simulink model "Speed_Control_Of_Induction_Motor_SVPWM"  (R2023b)
settings: Solver=ode3  StartTime=0.0  StopTime=100  FixedStep=1e-5  RelTol=1e-3
undefined symbols (not defined in the file): DiscIntNeverNeededParam
libraries: spsIGBTDiodeLib x6, spsCurrentMeasurementLib x3, spsAsynchronousMachineSIUnitsLib x1, slpidlib x1, simulink x1, spsDCVoltageSourceLib x1, sps_lib x1
settings Model: Creator=mailb  LastModifiedBy=mailb

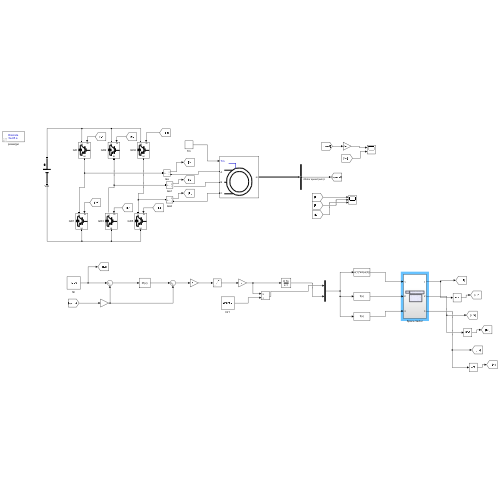
[thumbnail: Simulink's stored preview of the top-level diagram]
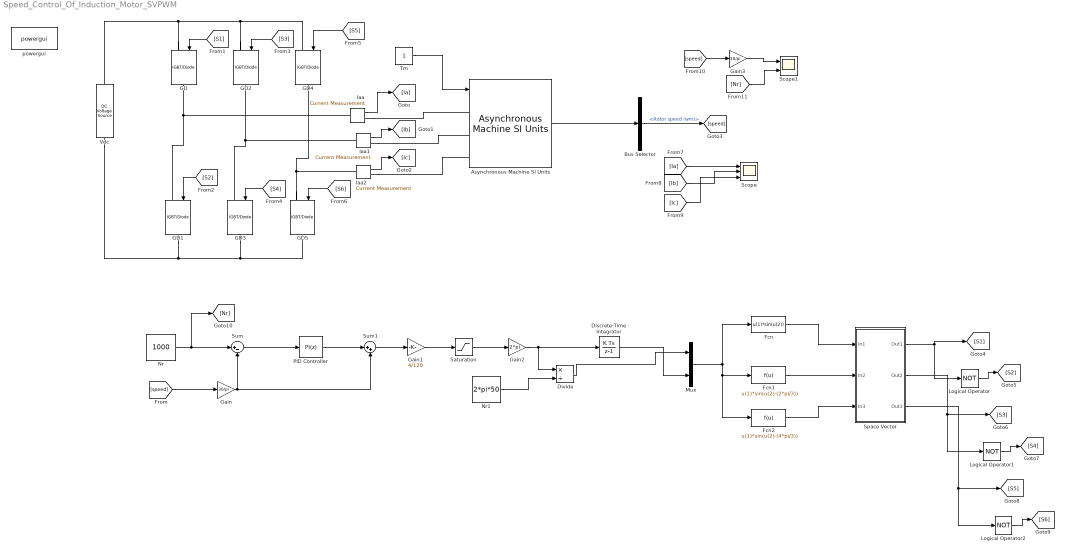
== system Speed_Control_Of_Induction_Motor_SVPWM ==
  Asynchronous Machine SI Units : spsAsynchronousMachineSIUnitsLib/Asynchronous Machine SI Units  RotorType=Squirrel-cage  PresetModel=No  MechanicalLoad=Torque Tm  ShowDetailedParameters=on  ReferenceFrame=Rotor  Units=SI  MeasurementBus=off  NominalParameters=[1.845e+04 400 50]  VoltageRatio=1  Stator=[0.5968 0.0003495]  Rotor=[0.6258 0.005473]  Cage1=[0.4155 0.002066]  Cage2=[0.4168 0.0003495]  Lm=0.0354  Mechanical=[0.05 0.005879 2]  PolePairs=2  InitialConditions=[0 0 0 0 0 0 0 0]  SimulateSaturation=off  Saturation=[14.03593122, 27.81365428, 53.79336849, 72.68890987, 97.98006896, 148.6815601, 215.7428561, 302.9841135, 428.7778367 ; 230, 322, 414, 460, 506, 552, 598, 644, 690]  LoadFlowParameters=1492000  TsPowergui=0  TsBlock=-1  IterativeModel=Trapezoidal non iterative  IterativeDiscreteModel=Trapezoidal non iterative  Pmec=1.492e+006
  Bus Selector : BusSelector  OutputSignals=Mechanical.Rotor speed (wm)
  Discrete-Time Integrator : DiscreteIntegrator  SampleTime=-1  ICPrevOutput=DiscIntNeverNeededParam  ICPrevScaledInput=DiscIntNeverNeededParam
  Divide : Product  Inputs=*/
  Fcn : Fcn  Expr=u(1)*sin(u(2))
  Fcn1 : Fcn  Expr=u(1)*sin(u(2)-(2*pi/3))
  Fcn2 : Fcn  Expr=u(1)*sin(u(2)-(4*pi/3))
  GD{,1..5} (6 alike) : spsIGBTDiodeLib/IGBT//Diode  Ron=1e-3  Rs=1e5  Cs=inf  Measurements=off
  Gain : Gain  Gain=30/pi
  Gain1 : Gain  Gain=4/120
  Gain2 : Gain  Gain=2*pi
  Gain3 : Gain  Gain=30/pi
  Iaa : spsCurrentMeasurementLib/Current Measurement  PhasorSimulation=off  OutputType=Complex  PSBequivalent=0
  Iaa1 : spsCurrentMeasurementLib/Current Measurement  PhasorSimulation=off  OutputType=Complex  PSBequivalent=0
  Iaa2 : spsCurrentMeasurementLib/Current Measurement  PhasorSimulation=off  OutputType=Complex  PSBequivalent=0
  Logical Operator : Logic  Operator=NOT  AllPortsSameDT=off  OutDataTypeStr=boolean
  Logical Operator1 : Logic  Operator=NOT  AllPortsSameDT=off  OutDataTypeStr=boolean
  Logical Operator2 : Logic  Operator=NOT  AllPortsSameDT=off  OutDataTypeStr=boolean
  Mux : Mux  Inputs=2
  Nr : Constant  Value=1000
  Nr1 : Constant  Value=2*pi*50
  PID Controller : slpidlib/PID Controller  Controller=PI  Form=Parallel  TimeDomain=Discrete-time  UseExternalTs=off  SampleTime=-1  IntegratorMethod=Forward Euler  FilterMethod=Forward Euler  ControllerParametersSource=internal  P=1  I=10  UseKiTs=off  D=0  N=100  UseFilter=on  TunerSelectOption=Transfer Function Based (PID Tuner App)  InitialConditionSource=internal  InitialConditionForIntegrator=0  InitialConditionForFilter=0  DifferentiatorICPrevScaledInput=0  ExternalReset=none  TrackingMode=off  Kt=1  LimitOutput=off  SatLimitsSource=internal  UpperSaturationLimit=inf  LowerSaturationLimit=-inf  LinearizeAsGain=on  AntiWindupMode=none  Kb=1  LimitIntegrator=off  UpperIntegratorSaturationLimit=inf  LowerIntegratorSaturationLimit=-inf  POutMin=[]  POutMax=[]  IOutMin=[]  IOutMax=[]  DOutMin=[]  DOutMax=[]  NOutMin=[]  NOutMax=[]  SumOutMin=[]  SumOutMax=[]  SaturationOutMin=[]  SaturationOutMax=[]  PParamMin=[]  PParamMax=[]  IParamMin=[]  IParamMax=[]  DParamMin=[]  DParamMax=[]  NParamMin=[]  NParamMax=[]  KbParamMin=[]  KbParamMax=[]  KtParamMin=[]  KtParamMax=[]  KbOutMin=[]  KbOutMax=[]  KtOutMin=[]  KtOutMax=[]  IntegratorOutMin=[]  IntegratorOutMax=[]  FilterOutMin=[]  FilterOutMax=[]  SumI1OutMin=[]  SumI1OutMax=[]  SumI2OutMin=[]  SumI2OutMax=[]  SumI3OutMin=[]  SumI3OutMax=[]  SumI4OutMin=[]  SumI4OutMax=[]  SumDOutMin=[]  SumDOutMax=[]  DifferentiatorOutMin=[]  DifferentiatorOutMax=[]  FilterDiffOutCoefMin=[]  FilterDiffOutCoefMax=[]  ReciprocalOutMin=[]  ReciprocalOutMax=[]  SumDenOutMin=[]  SumDenOutMax=[]  SumNumOutMin=[]  SumNumOutMax=[]  DivideOutMin=[]  DivideOutMax=[]  UdiffTsProdOutMin=[]  UdiffTsProdOutMax=[]  NTsProdOutMin=[]  NTsProdOutMax=[]  UintegralTsProdOutMin=[]  UintegralTsProdOutMax=[]  UngainTsProdOutMin=[]  UngainTsProdOutMax=[]  ClampingZeroOutDataTypeStr=Inherit: Inherit via back propagation  ClampingZeroOutMin=[]  ClampingZeroOutMax=[]  FilterDenConstantOutDataTypeStr=Inherit: Inherit via back propagation  FilterDenConstantOutMin=[]  FilterDenConstantOutMax=[]  PCopyOutDataTypeStr=Inherit: Inherit via back propagation  PCopyOutMin=[]  PCopyOutMax=[]  NCopyOutDataTypeStr=Inherit: Inherit via back propagation  NCopyOutMin=[]  NCopyOutMax=[]  IntegratorContinuousStateAttributes=''  IntegratorStateMustResolveToSignalObject=off  IntegratorRTWStateStorageClass=Auto  FilterContinuousStateAttributes=''  FilterStateMustResolveToSignalObject=off  FilterRTWStateStorageClass=Auto  ParallelPVariant=InternalParameters  IdealPVariant=Disabled  IVariant=InternalParameters  DVariant=Disabled  IntegratorVariant=Discrete  SatVariant=Disabled  AWVariant=Passthrough  PCopyVariant=Disabled  TRVariant=Disabled  FdbkBlocksVariant=Forward  IdealPFdbkVariant=Disabled  SatFdbkVariant=Disabled  DerivativeFilterVariant=Disabled  NVariant=Disabled  NCopyVariant=Disabled_SignalSpec  FilterICVariant=Disabled  IntegratorICVariant=InternalICs  ExternalResetVariant=Disabled  TRSumVariant=Passthrough  SumFdbkVariant=Disabled  SumVariant=Sum_PI  TsampFilterVariant=InternalTs  TsampNgainVariant=Passthrough  TsampIntegralVariant=Disabled_SignalSpec  ExternalSaturationOutDataTypeStr=Inherit: Same as second input
  Saturation : Saturate  UpperLimit=50  LowerLimit=0
  Scope : Scope  NumInputPorts=3
  Scope1 : Scope  NumInputPorts=2
  Space Vector : Subsystem
  Sum : Sum  Inputs=|+-
  Sum1 : Sum  Inputs=|++
  Tm : Constant
  Vdc : spsDCVoltageSourceLib/DC Voltage Source  Amplitude=572  Measurements=None
  powergui : sps_lib/powergui  Priority=1  SimulationMode=Discrete  SampleTime=50e-6  frequency=60  Iterations=50  frequencyindice=50  Pbase=100e6  ErrMax=1e-4  UnitsV=kV  UnitsW=MW  buscounter=0  FunctionMessages=off  echomessages=off  EnableUseOfTLC=off  CurrentSourceSwitches=off  DisableSnubberDevices=off  DisableRonSwitches=off  DisableVfSwitches=off  DisplayEquations=off  AutomaticDiscreteSolvers=off  SolverType=Tustin/Backward Euler (TBE)  Interpol=off  ExternalGateDelay=off  methode=off  Ts=100  x0status=blocks  SPID=on  SwTol=0  HookPort=off  NonlinearTolerance=1e-4  nMaxIteration=100  ContinueOnMaxIteration=off  RestoreLinks=warning  ResistiveCurrentMeasurement=off  Frange=[0:2:500]  Ylog=off  Xlog=on  ShowGrid=off  save=off  variable=ZData  structure=0  ZoomFFT=off  StartTime=0.0  cycles=1  DisplayStyle=1  fundamental=60  FreqAxis=off  MaxFrequency=1000  frequencyindicesteady=1  RmsSteady=1  display=off
  wires:
  Iaa/1 -> [Ia]
  Iaa1/1 -> [Ib]
  Iaa2/1 -> [Ic]
  Tm/1 -> Asynchronous Machine SI Units/1
  Asynchronous Machine SI Units/1 -> Bus Selector/1
  Bus Selector/1 -> [speed]  "<Rotor speed (wm)>"
  Nr/1 -> [Nr], Sum/1
  [speed] -> Gain/1
  Gain/1 -> Sum/2, Sum1/2
  Sum/1 -> PID Controller/1
  PID Controller/1 -> Sum1/1
  Sum1/1 -> Gain1/1
  Gain1/1 -> Saturation/1
  Saturation/1 -> Gain2/1
  Gain2/1 -> Discrete-Time Integrator/1, Divide/1
  Nr1/1 -> Divide/2
  Discrete-Time Integrator/1 -> Mux/2
  Divide/1 -> Mux/1
  Mux/1 -> Fcn2/1, Fcn1/1, Fcn/1
  Fcn/1 -> Space Vector/1(In1)
  Fcn1/1 -> Space Vector/2(In2)
  Fcn2/1 -> Space Vector/3(In3)
  Space Vector/1(Out1) -> [S1], Logical Operator/1
  Logical Operator/1 -> [S2]
  Logical Operator1/1 -> [S4]
  Space Vector/2(Out2) -> Logical Operator1/1, [S3]
  Logical Operator2/1 -> [S6]
  Space Vector/3(Out3) -> Logical Operator2/1, [S5]
  [S1] -> GD/1
  [S2] -> GD1/1
  [S3] -> GD2/1
  [S4] -> GD3/1
  [S5] -> GD4/1
  [S6] -> GD5/1
  [Ia] -> Scope/1
  [Ib] -> Scope/2
  [Ic] -> Scope/3
  [Nr] -> Scope1/2
  [speed] -> Gain3/1
  Gain3/1 -> Scope1/1
  connections:
  GD1/LConn1 -- Iaa/LConn1 -- GD/RConn1
  GD3/LConn1 -- Iaa1/LConn1 -- GD2/RConn1
  GD5/LConn1 -- Iaa2/LConn1 -- GD4/RConn1
  GD/LConn1 -- Vdc/RConn1 -- GD2/LConn1 -- GD4/LConn1
  GD1/RConn1 -- Vdc/LConn1 -- GD3/RConn1 -- GD5/RConn1
  Iaa/RConn1 -- Asynchronous Machine SI Units/LConn1
  Iaa1/RConn1 -- Asynchronous Machine SI Units/LConn2
  Iaa2/RConn1 -- Asynchronous Machine SI Units/LConn3

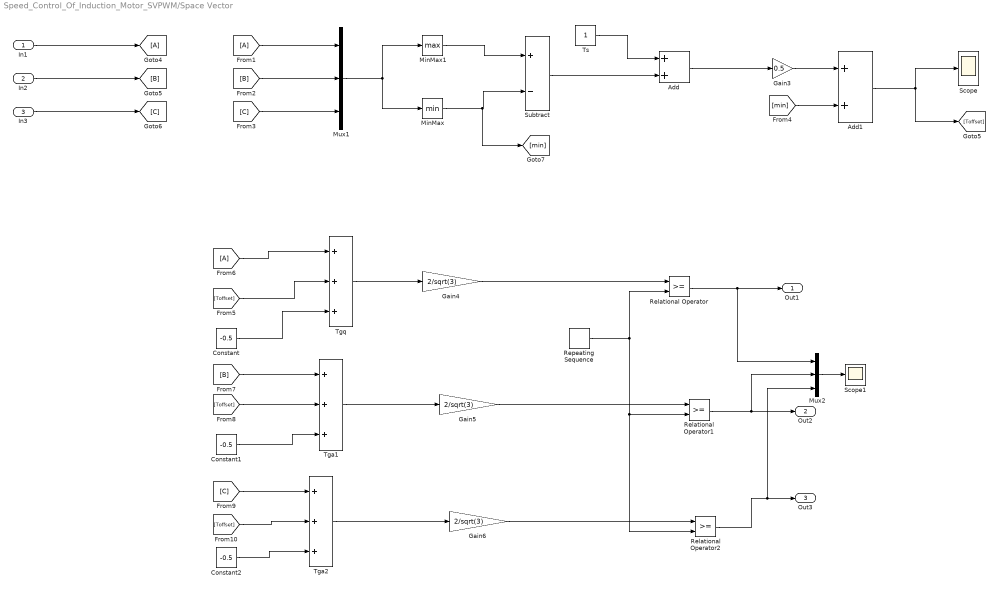
== system Speed_Control_Of_Induction_Motor_SVPWM/Space Vector ==
  In1 : Inport
  In2 : Inport  Port=2
  In3 : Inport  Port=3
  Add : Sum
  Add1 : Sum
  Constant : Constant  Value=-0.5
  Constant1 : Constant  Value=-0.5
  Constant2 : Constant  Value=-0.5
  From1 : From
  From6 : From
  Gain3 : Gain  Gain=0.5
  Gain4 : Gain  Gain=2/sqrt(3)
  Gain5 : Gain  Gain=2/sqrt(3)
  Gain6 : Gain  Gain=2/sqrt(3)
  Goto4 : Goto
  MinMax : MinMax
  MinMax1 : MinMax  Function=max
  Mux1 : Mux  Inputs=3
  Mux2 : Mux  Inputs=3
  Relational Operator : RelationalOperator  OutDataTypeStr=boolean  RndMeth=Simplest  InputSameDT=off
  Relational Operator1 : RelationalOperator  OutDataTypeStr=boolean  RndMeth=Simplest  InputSameDT=off
  Relational Operator2 : RelationalOperator  OutDataTypeStr=boolean  RndMeth=Simplest  InputSameDT=off
  Repeating Sequence : simulink/Sources/Repeating Sequence  rep_seq_t=[0 0.01]  rep_seq_y=[0 0.01]
  Scope : Scope
  Scope1 : Scope
  Subtract : Sum  Inputs=+-
  Tga1 : Sum  Inputs=+++
  Tga2 : Sum  Inputs=+++
  Tgq : Sum  Inputs=+++
  Ts : Constant
  Out1 : Outport
  Out2 : Outport  Port=2
  Out3 : Outport  Port=3
  wires:
  Gain5/1 -> Relational Operator1/1
  From1/1 -> Mux1/1
  From6/1 -> Tgq/1
  Tga1/1 -> Gain5/1
  Constant/1 -> Tgq/3
  Constant2/1 -> Tga2/3
  Add1/1 -> Scope/1, [Toffset]
  [C] -> Mux1/3
  Add/1 -> Gain3/1
  Mux1/1 -> MinMax/1, MinMax1/1
  Repeating Sequence/1 -> Relational Operator2/2, Relational Operator1/2, Relational Operator/2
  [Toffset] -> Tga2/2
  Relational Operator2/1 -> Out3/1, Mux2/3
  [B] -> Tga1/1
  Subtract/1 -> Add/2
  Tgq/1 -> Gain4/1
  Gain4/1 -> Relational Operator/1
  MinMax1/1 -> Subtract/1
  [B] -> Mux1/2
  [Toffset] -> Tga1/2
  In3/1 -> [C]
  Gain6/1 -> Relational Operator2/1
  Relational Operator/1 -> Out1/1, Mux2/1
  [Toffset] -> Tgq/2
  In2/1 -> [B]
  Constant1/1 -> Tga1/3
  Gain3/1 -> Add1/1
  [C] -> Tga2/1
  MinMax/1 -> [min], Subtract/2
  Tga2/1 -> Gain6/1
  Relational Operator1/1 -> Out2/1, Mux2/2
  [min] -> Add1/2
  Ts/1 -> Add/1
  Mux2/1 -> Scope1/1
  In1/1 -> Goto4/1
